simulink model "full_correlator"  (R2022a)
settings: Solver=VariableStepDiscrete  StartTime=0.0  StopTime=4000  RelTol=1e-3
libraries: hdlBasic x2638, hdlSSR x215, hdlDSPIP x4, xbsIndex_r4 x1, xps_library x1
(part 32 of 43)

== system full_correlator/Subsystem5/Vector Complex Mult2/Mult6 ==
  note: MULT2 and MULT3 settings
      | -------------------------------------
      | w mux = 0 op[8:7] = 00
      | z mux = C op[6:4] = 011
      | x mux = M op[3:2] = 01
      | y mux = M op[1:0] = 01
      | carryinsel = 000
      | inmode = bin2dec('00100') (D+B) vs bin2dec('01100') (D-B);
      | inmode[4]=0 for B2 selection; inmode[3]=0 preadd; inmode[0]=0 A2
      | alumode = bin2dec('0000') (Z+W+X+Y+CIN)
  note: latency = 6
  note: -(D-A)*B
  note: A*B
      | a = 30 bits
      | b = 18 bits,
      | d = 27 bits
  note: (A_re[25:0] + jA_im[25:0]) x (B_re[16:0] + jB_im[16:0])= Out_re[43:0] + jOut_im[43:0]
      | –Out_re[43:0]= ((A_re[25:0] x B_re[16:0]) - (A_im[25:0] x B_im[16:0]))
      | –Out_im[43:0]= ((A_re[25:0] x B_im[16:0]) + (A_im[25:0] x B_re[16:0]))
      |
      | Re-factored for three DSP slice version that uses PreAdders
      | –Out_re[43:0]= (CF) - ((B_re[16:0] – B_im[16:0]) x A_re[25:0])
      | –Out_im[43:0]= (CF) + ((B_re[16:0] + B_im[16:0]) x A_im[25:0])
      | Common factor that is shared
      | –CF=((A_re[25:0] – A_im[25:0]) x B_im[16:0])
  note: MULT1 settings
      | -------------------------------------
      | w mux = rnd op[8:7] = 00
      | z mux = C op[6:4] = 000
      | x mux = M op[3:2] = 01
      | y mux = M op[1:0] = 01
      | carryinsel = 000
      | inmode = bin2dec('01101') (D-A)
      | inmode[4]=0 for B2 selection; inmode[3]=0 preadd; inmode[0]=0 A2
      | alumode = bin2dec('0011') Z-(W+X+Y+CIN)
  note: (D-B)*A+C
  note: (D+B)*A+C
  A_re : Inport
  A_im : Inport  Port=2
  B_re : Inport  Port=3
  B_im : Inport  Port=4
  BitBasher : hdlBasic/BitBasher  bitexpr=out_44_40={in_48[43:0]}  display_expr=off  sr_1=out_44_40  arith_type1="Signed  (2's comp)"  bin_pt1=41  sr_2=2  arith_type2=Unsigned  bin_pt2=0  sr_3=3  arith_type3=Unsigned  bin_pt3=0  sr_4=4  arith_type4=Unsigned  bin_pt4=0  XmcBlockStatus=1  maskContainerNames=group1  block_type=bitbasher  block_config=sysgen:BitBasher_config
  BitBasher1 : hdlBasic/BitBasher  bitexpr=out_44_40={in_48[43:0]}  display_expr=off  sr_1=out_44_40  arith_type1="Signed  (2's comp)"  bin_pt1=41  sr_2=2  arith_type2=Unsigned  bin_pt2=0  sr_3=3  arith_type3=Unsigned  bin_pt3=0  sr_4=4  arith_type4=Unsigned  bin_pt4=0  XmcBlockStatus=1  maskContainerNames=group1  block_type=bitbasher  block_config=sysgen:BitBasher_config
  Constant10 : hdlBasic/Constant  const=bin2dec('000')  gui_display_data_type=Fixed-point  arith_type=Unsigned  n_bits=3  bin_pt=0  preci_type=Single  exp_width=8  frac_width=24  explicit_period=off  period=1  XmcBlockStatus=1  maskContainerNames=tabcontainer1  block_type=constant  block_config=sysgen:Constant_config
  Constant11 : hdlBasic/Constant  const=bin2dec('01101')  gui_display_data_type=Fixed-point  arith_type=Unsigned  n_bits=5  bin_pt=0  preci_type=Single  exp_width=8  frac_width=24  explicit_period=off  period=1  XmcBlockStatus=1  maskContainerNames=tabcontainer1  block_type=constant  block_config=sysgen:Constant_config
  Constant12 : hdlBasic/Constant  const=bin2dec('000000101')  gui_display_data_type=Fixed-point  arith_type=Unsigned  n_bits=9  bin_pt=0  preci_type=Single  exp_width=8  frac_width=24  explicit_period=off  period=1  XmcBlockStatus=1  maskContainerNames=tabcontainer1  block_type=constant  block_config=sysgen:Constant_config
  Constant13 : hdlBasic/Constant  const=0  gui_display_data_type=Fixed-point  arith_type=Unsigned  n_bits=1  bin_pt=0  preci_type=Single  exp_width=8  frac_width=24  explicit_period=off  period=1  XmcBlockStatus=1  maskContainerNames=tabcontainer1  block_type=constant  block_config=sysgen:Constant_config
  Constant14 : hdlBasic/Constant  const=0  gui_display_data_type=Fixed-point  arith_type=Unsigned  n_bits=1  bin_pt=0  preci_type=Single  exp_width=8  frac_width=24  explicit_period=off  period=1  XmcBlockStatus=1  maskContainerNames=tabcontainer1  block_type=constant  block_config=sysgen:Constant_config
  Constant15 : hdlBasic/Constant  const=bin2dec('000')  gui_display_data_type=Fixed-point  arith_type=Unsigned  n_bits=3  bin_pt=0  preci_type=Single  exp_width=8  frac_width=24  explicit_period=off  period=1  XmcBlockStatus=1  maskContainerNames=tabcontainer1  block_type=constant  block_config=sysgen:Constant_config
  Constant16 : hdlBasic/Constant  const=bin2dec('00100')  gui_display_data_type=Fixed-point  arith_type=Unsigned  n_bits=5  bin_pt=0  preci_type=Single  exp_width=8  frac_width=24  explicit_period=off  period=1  XmcBlockStatus=1  maskContainerNames=tabcontainer1  block_type=constant  block_config=sysgen:Constant_config
  Constant17 : hdlBasic/Constant  const=bin2dec('000110101')  gui_display_data_type=Fixed-point  arith_type=Unsigned  n_bits=9  bin_pt=0  preci_type=Single  exp_width=8  frac_width=24  explicit_period=off  period=1  XmcBlockStatus=1  maskContainerNames=tabcontainer1  block_type=constant  block_config=sysgen:Constant_config
  Constant18 : hdlBasic/Constant  const=bin2dec('0000')  gui_display_data_type=Fixed-point  arith_type=Unsigned  n_bits=4  bin_pt=0  preci_type=Single  exp_width=8  frac_width=24  explicit_period=off  period=1  XmcBlockStatus=1  maskContainerNames=tabcontainer1  block_type=constant  block_config=sysgen:Constant_config
  Constant4 : hdlBasic/Constant  const=bin2dec('000')  gui_display_data_type=Fixed-point  arith_type=Unsigned  n_bits=3  bin_pt=0  preci_type=Single  exp_width=8  frac_width=24  explicit_period=off  period=1  XmcBlockStatus=1  maskContainerNames=tabcontainer1  block_type=constant  block_config=sysgen:Constant_config
  Constant5 : hdlBasic/Constant  const=bin2dec('01100')  gui_display_data_type=Fixed-point  arith_type=Unsigned  n_bits=5  bin_pt=0  preci_type=Single  exp_width=8  frac_width=24  explicit_period=off  period=1  XmcBlockStatus=1  maskContainerNames=tabcontainer1  block_type=constant  block_config=sysgen:Constant_config
  Constant6 : hdlBasic/Constant  const=bin2dec('000110101')  gui_display_data_type=Fixed-point  arith_type=Unsigned  n_bits=9  bin_pt=0  preci_type=Single  exp_width=8  frac_width=24  explicit_period=off  period=1  XmcBlockStatus=1  maskContainerNames=tabcontainer1  block_type=constant  block_config=sysgen:Constant_config
  Constant7 : hdlBasic/Constant  const=bin2dec('0000')  gui_display_data_type=Fixed-point  arith_type=Unsigned  n_bits=4  bin_pt=0  preci_type=Single  exp_width=8  frac_width=24  explicit_period=off  period=1  XmcBlockStatus=1  maskContainerNames=tabcontainer1  block_type=constant  block_config=sysgen:Constant_config
  Constant8 : hdlBasic/Constant  const=bin2dec('0011')  gui_display_data_type=Fixed-point  arith_type=Unsigned  n_bits=4  bin_pt=0  preci_type=Single  exp_width=8  frac_width=24  explicit_period=off  period=1  XmcBlockStatus=1  maskContainerNames=tabcontainer1  block_type=constant  block_config=sysgen:Constant_config
  Constant9 : hdlBasic/Constant  const=0  gui_display_data_type=Fixed-point  arith_type=Unsigned  n_bits=1  bin_pt=0  preci_type=Single  exp_width=8  frac_width=24  explicit_period=off  period=1  XmcBlockStatus=1  maskContainerNames=tabcontainer1  block_type=constant  block_config=sysgen:Constant_config
  Delay : hdlBasic/Delay  rst=off  en=off  latency=2  reg_retiming=off  XmcBlockStatus=1  maskContainerNames=group1  block_type=delay  block_config=sysgen:Delay_config
  Delay1 : hdlBasic/Delay  rst=off  en=off  latency=2  reg_retiming=off  XmcBlockStatus=1  maskContainerNames=group1  block_type=delay  block_config=sysgen:Delay_config
  MULT1 : hdlBasic/DSP48E2   use_a=Direct from a port  use_b=Direct from b port  addsub_mode=One 48-bit Unit  xl_useadderonly=off  xl_dynamicmult=off  preaddinsel=A  amultsel=AD  bmultsel=B  enable_d=on  reset_preg=off  auto_reset_pr=RESET  pattern_from_creg=Pattern Input from c port  pattern='000000000000'  mask_from_creg=Mask Input from c port  pattern_mask='000000000000'  rnd='000000000000'  widexor=off  xormode=XOR12  use_op=off  use_creg=off  rst_all=off  en_all=off  use_pcin=off  use_carrycascin=off  use_multsignin=off  use_carryout=off  use_patterndetect=off  use_patternbdetect=off  use_overflow=off  use_underflow=off  use_acout=on  use_bcout=on  use_pcout=off  use_multsignout=off  use_carrycascout=off  pipeline_a=2  pipeline_b=2  pipeline_acout=2  pipeline_bcout=1  pipeline_c=on  pipeline_p=on  pipeline_mult=on  pipeline_opmode=off  pipeline_alumode=off  pipeline_carryin=off  pipeline_carryinsel=off  dreg=on  adreg=on  register_inmode=off  rst_a=off  rst_b=off  rst_c=off  rst_mult=off  rst_p=off  rst_carry_in=off  rst_alumode=off  rst_ctrl=off  reset_port_d=off  reset_port_inmode=off  en_a1=off  en_a2=off  en_b1=off  en_b2=off  en_c=off  en_mult=off  en_p=off  en_carry_in=off  en_alumode=off  en_multcarryin=off  en_ctrl=off  enable_port_regd=off  enable_port_regad=off  enable_port_reginmode=off  alumode_inverted=off  alumode_inverted_value='0000'  is_carryin_inverted=off  inmode_inverted=off  inmode_inverted_value='00000'  opmode_inverted=off  opmode_inverted_value='000000000'  is_rstallcarryin_inverted=off  is_rstalumode_inverted=off  is_rsta_inverted=off  is_rstb_inverted=off  is_rstc_inverted=off  is_rstd_inverted=off  is_rstctrl_inverted=off  is_rstinmode_inverted=off  is_rstm_inverted=off  is_rstp_inverted=off  use_synth_model=off  simulation_type=fast_sim  is_clk_inverted=false  XmcBlockStatus=1  maskContainerNames=tabcontainer1  block_type=dsp48e2  block_config=sysgen:DSP48E2_config  block_height=1080  block_width=800
  MULT2 : hdlBasic/DSP48E2   use_a=Cascaded from acin port  use_b=Cascaded from bcin port  addsub_mode=One 48-bit Unit  xl_useadderonly=off  xl_dynamicmult=off  preaddinsel=B  amultsel=A  bmultsel=AD  enable_d=on  reset_preg=off  auto_reset_pr=RESET  pattern_from_creg=Pattern Input from c port  pattern='000000000000'  mask_from_creg=Mask Input from c port  pattern_mask='000000000000'  rnd='000000000000'  widexor=off  xormode=XOR12  use_op=off  use_creg=on  rst_all=off  en_all=off  use_pcin=off  use_carrycascin=off  use_multsignin=off  use_carryout=off  use_patterndetect=off  use_patternbdetect=off  use_overflow=off  use_underflow=off  use_acout=off  use_bcout=on  use_pcout=off  use_multsignout=off  use_carrycascout=off  pipeline_a=2  pipeline_b=2  pipeline_acout=1  pipeline_bcout=1  pipeline_c=on  pipeline_p=on  pipeline_mult=on  pipeline_opmode=off  pipeline_alumode=off  pipeline_carryin=off  pipeline_carryinsel=off  dreg=on  adreg=on  register_inmode=off  rst_a=off  rst_b=off  rst_c=off  rst_mult=off  rst_p=off  rst_carry_in=off  rst_alumode=off  rst_ctrl=off  reset_port_d=off  reset_port_inmode=off  en_a1=off  en_a2=off  en_b1=off  en_b2=off  en_c=off  en_mult=off  en_p=off  en_carry_in=off  en_alumode=off  en_multcarryin=off  en_ctrl=off  enable_port_regd=off  enable_port_regad=off  enable_port_reginmode=off  alumode_inverted=off  alumode_inverted_value='0000'  is_carryin_inverted=off  inmode_inverted=off  inmode_inverted_value='00000'  opmode_inverted=off  opmode_inverted_value='000000000'  is_rstallcarryin_inverted=off  is_rstalumode_inverted=off  is_rsta_inverted=off  is_rstb_inverted=off  is_rstc_inverted=off  is_rstd_inverted=off  is_rstctrl_inverted=off  is_rstinmode_inverted=off  is_rstm_inverted=off  is_rstp_inverted=off  use_synth_model=off  simulation_type=fast_sim  is_clk_inverted=false  XmcBlockStatus=1  maskContainerNames=tabcontainer1  block_type=dsp48e2  block_config=sysgen:DSP48E2_config  block_height=1080  block_width=800
  MULT3 : hdlBasic/DSP48E2   use_a=Direct from a port  use_b=Cascaded from bcin port  addsub_mode=One 48-bit Unit  xl_useadderonly=off  xl_dynamicmult=off  preaddinsel=B  amultsel=A  bmultsel=AD  enable_d=on  reset_preg=off  auto_reset_pr=RESET  pattern_from_creg=Pattern Input from c port  pattern='000000000000'  mask_from_creg=Mask Input from c port  pattern_mask='000000000000'  rnd='000000000000'  widexor=off  xormode=XOR12  use_op=off  use_creg=on  rst_all=off  en_all=off  use_pcin=off  use_carrycascin=off  use_multsignin=off  use_carryout=off  use_patterndetect=off  use_patternbdetect=off  use_overflow=off  use_underflow=off  use_acout=off  use_bcout=off  use_pcout=off  use_multsignout=off  use_carrycascout=off  pipeline_a=2  pipeline_b=1  pipeline_acout=1  pipeline_bcout=1  pipeline_c=on  pipeline_p=on  pipeline_mult=on  pipeline_opmode=off  pipeline_alumode=off  pipeline_carryin=off  pipeline_carryinsel=off  dreg=on  adreg=on  register_inmode=off  rst_a=off  rst_b=off  rst_c=off  rst_mult=off  rst_p=off  rst_carry_in=off  rst_alumode=off  rst_ctrl=off  reset_port_d=off  reset_port_inmode=off  en_a1=off  en_a2=off  en_b1=off  en_b2=off  en_c=off  en_mult=off  en_p=off  en_carry_in=off  en_alumode=off  en_multcarryin=off  en_ctrl=off  enable_port_regd=off  enable_port_regad=off  enable_port_reginmode=off  alumode_inverted=off  alumode_inverted_value='0000'  is_carryin_inverted=off  inmode_inverted=off  inmode_inverted_value='00000'  opmode_inverted=off  opmode_inverted_value='000000000'  is_rstallcarryin_inverted=off  is_rstalumode_inverted=off  is_rsta_inverted=off  is_rstb_inverted=off  is_rstc_inverted=off  is_rstd_inverted=off  is_rstctrl_inverted=off  is_rstinmode_inverted=off  is_rstm_inverted=off  is_rstp_inverted=off  use_synth_model=off  simulation_type=fast_sim  is_clk_inverted=false  XmcBlockStatus=1  maskContainerNames=tabcontainer1  block_type=dsp48e2  block_config=sysgen:DSP48E2_config  block_height=1080  block_width=800
  bit_bash1 : hdlBasic/BitBasher  bitexpr=ao={ain[25],ain[25:0]} % sign extend to 27 bits  display_expr=off  sr_1=ao  arith_type1="Signed  (2's comp)"  bin_pt1=0  sr_2=a_dsp48  arith_type2="Signed  (2's comp)"  bin_pt2=0  sr_3=p2  arith_type3=Unsigned  bin_pt3=0  sr_4=4  arith_type4=Unsigned  bin_pt4=0  XmcBlockStatus=1  maskContainerNames=group1  block_type=bitbasher  block_config=sysgen:BitBasher_config
  bit_bash2 : hdlBasic/BitBasher  bitexpr=ao={4{ain[25]},ain[25:0]} % sign extend to 30 bits  display_expr=off  sr_1=ao  arith_type1="Signed  (2's comp)"  bin_pt1=0  sr_2=a_dsp48  arith_type2="Signed  (2's comp)"  bin_pt2=0  sr_3=p2  arith_type3=Unsigned  bin_pt3=0  sr_4=4  arith_type4=Unsigned  bin_pt4=0  XmcBlockStatus=1  maskContainerNames=group1  block_type=bitbasher  block_config=sysgen:BitBasher_config
  bit_bash3 : hdlBasic/BitBasher  bitexpr=bo={ bin[16] , bin[16:0] }; % sign extend to 18 bit data  display_expr=off  sr_1=bo  arith_type1="Signed  (2's comp)"  bin_pt1=0  sr_2=b_dsp48  arith_type2="Signed  (2's comp)"  bin_pt2=0  sr_3=p2  arith_type3=Unsigned  bin_pt3=0  sr_4=4  arith_type4=Unsigned  bin_pt4=0  XmcBlockStatus=1  maskContainerNames=group1  block_type=bitbasher  block_config=sysgen:BitBasher_config
  bit_bash4 : hdlBasic/BitBasher  bitexpr=bo={ 10{bin[16]} , bin[16:0] }; % sign extend to 27 bit data  display_expr=off  sr_1=bo  arith_type1="Signed  (2's comp)"  bin_pt1=0  sr_2=b_dsp48  arith_type2="Signed  (2's comp)"  bin_pt2=0  sr_3=p2  arith_type3=Unsigned  bin_pt3=0  sr_4=4  arith_type4=Unsigned  bin_pt4=0  XmcBlockStatus=1  maskContainerNames=group1  block_type=bitbasher  block_config=sysgen:BitBasher_config
  bit_bash8 : hdlBasic/BitBasher  bitexpr=ao={3{ain[26]},ain[26:0]} % sign extend to 30 bits  display_expr=off  sr_1=ao  arith_type1="Signed  (2's comp)"  bin_pt1=0  sr_2=a_dsp48  arith_type2="Signed  (2's comp)"  bin_pt2=0  sr_3=p2  arith_type3=Unsigned  bin_pt3=0  sr_4=4  arith_type4=Unsigned  bin_pt4=0  XmcBlockStatus=1  maskContainerNames=group1  block_type=bitbasher  block_config=sysgen:BitBasher_config
  C_re : Outport  VectorParamsAs1DForOutWhenUnconnected=off
  C_im : Outport  Port=2  VectorParamsAs1DForOutWhenUnconnected=off
  wires:
  BitBasher1/1 -> C_re/1  "C_re"
  MULT3/1 -> BitBasher/1
  Delay/1 -> MULT3/4, MULT2/4  "B_re_int_dly2"
  Constant15/1 -> MULT3/8
  MULT1/3 -> MULT2/2  "bcout_MULT1"
  Constant7/1 -> MULT2/6
  Constant13/1 -> MULT2/7
  Constant4/1 -> MULT2/8
  Constant5/1 -> MULT2/9
  Constant8/1 -> MULT1/5
  Constant9/1 -> MULT1/6
  Delay1/1 -> MULT3/1  "A_im_int_dly2"
  bit_bash4/1 -> Delay/1  "B_re_int"
  bit_bash8/1 -> Delay1/1
  Constant6/1 -> MULT2/5
  MULT2/2 -> MULT3/2  "bcout_MULT2"
  Constant18/1 -> MULT3/6
  Constant11/1 -> MULT1/8
  Constant12/1 -> MULT1/4
  Constant10/1 -> MULT1/7
  MULT1/2 -> MULT2/1  "acout_MULT1"
  MULT2/1 -> BitBasher1/1  "out_re"
  Constant16/1 -> MULT3/9
  Constant14/1 -> MULT3/7
  Constant17/1 -> MULT3/5
  A_im/1 -> bit_bash1/1
  B_im/1 -> bit_bash3/1
  A_re/1 -> bit_bash2/1
  MULT1/1 -> MULT3/3, MULT2/3  "common"
  bit_bash1/1 -> bit_bash8/1, MULT1/3  "A_im_int"
  bit_bash2/1 -> MULT1/1  "A_re_int"
  bit_bash3/1 -> MULT1/2  "B_im_int"
  B_re/1 -> bit_bash4/1
  BitBasher/1 -> C_im/1  "C_im"

== system full_correlator/Subsystem5/Vector Complex Mult2/Mult7 ==
  note: MULT2 and MULT3 settings
      | -------------------------------------
      | w mux = 0 op[8:7] = 00
      | z mux = C op[6:4] = 011
      | x mux = M op[3:2] = 01
      | y mux = M op[1:0] = 01
      | carryinsel = 000
      | inmode = bin2dec('00100') (D+B) vs bin2dec('01100') (D-B);
      | inmode[4]=0 for B2 selection; inmode[3]=0 preadd; inmode[0]=0 A2
      | alumode = bin2dec('0000') (Z+W+X+Y+CIN)
  note: latency = 6
  note: -(D-A)*B
  note: A*B
      | a = 30 bits
      | b = 18 bits,
      | d = 27 bits
  note: (A_re[25:0] + jA_im[25:0]) x (B_re[16:0] + jB_im[16:0])= Out_re[43:0] + jOut_im[43:0]
      | –Out_re[43:0]= ((A_re[25:0] x B_re[16:0]) - (A_im[25:0] x B_im[16:0]))
      | –Out_im[43:0]= ((A_re[25:0] x B_im[16:0]) + (A_im[25:0] x B_re[16:0]))
      |
      | Re-factored for three DSP slice version that uses PreAdders
      | –Out_re[43:0]= (CF) - ((B_re[16:0] – B_im[16:0]) x A_re[25:0])
      | –Out_im[43:0]= (CF) + ((B_re[16:0] + B_im[16:0]) x A_im[25:0])
      | Common factor that is shared
      | –CF=((A_re[25:0] – A_im[25:0]) x B_im[16:0])
  note: MULT1 settings
      | -------------------------------------
      | w mux = rnd op[8:7] = 00
      | z mux = C op[6:4] = 000
      | x mux = M op[3:2] = 01
      | y mux = M op[1:0] = 01
      | carryinsel = 000
      | inmode = bin2dec('01101') (D-A)
      | inmode[4]=0 for B2 selection; inmode[3]=0 preadd; inmode[0]=0 A2
      | alumode = bin2dec('0011') Z-(W+X+Y+CIN)
  note: (D-B)*A+C
  note: (D+B)*A+C
  A_re : Inport
  A_im : Inport  Port=2
  B_re : Inport  Port=3
  B_im : Inport  Port=4
  BitBasher : hdlBasic/BitBasher  bitexpr=out_44_40={in_48[43:0]}  display_expr=off  sr_1=out_44_40  arith_type1="Signed  (2's comp)"  bin_pt1=41  sr_2=2  arith_type2=Unsigned  bin_pt2=0  sr_3=3  arith_type3=Unsigned  bin_pt3=0  sr_4=4  arith_type4=Unsigned  bin_pt4=0  XmcBlockStatus=1  maskContainerNames=group1  block_type=bitbasher  block_config=sysgen:BitBasher_config
  BitBasher1 : hdlBasic/BitBasher  bitexpr=out_44_40={in_48[43:0]}  display_expr=off  sr_1=out_44_40  arith_type1="Signed  (2's comp)"  bin_pt1=41  sr_2=2  arith_type2=Unsigned  bin_pt2=0  sr_3=3  arith_type3=Unsigned  bin_pt3=0  sr_4=4  arith_type4=Unsigned  bin_pt4=0  XmcBlockStatus=1  maskContainerNames=group1  block_type=bitbasher  block_config=sysgen:BitBasher_config
  Constant10 : hdlBasic/Constant  const=bin2dec('000')  gui_display_data_type=Fixed-point  arith_type=Unsigned  n_bits=3  bin_pt=0  preci_type=Single  exp_width=8  frac_width=24  explicit_period=off  period=1  XmcBlockStatus=1  maskContainerNames=tabcontainer1  block_type=constant  block_config=sysgen:Constant_config
  Constant11 : hdlBasic/Constant  const=bin2dec('01101')  gui_display_data_type=Fixed-point  arith_type=Unsigned  n_bits=5  bin_pt=0  preci_type=Single  exp_width=8  frac_width=24  explicit_period=off  period=1  XmcBlockStatus=1  maskContainerNames=tabcontainer1  block_type=constant  block_config=sysgen:Constant_config
  Constant12 : hdlBasic/Constant  const=bin2dec('000000101')  gui_display_data_type=Fixed-point  arith_type=Unsigned  n_bits=9  bin_pt=0  preci_type=Single  exp_width=8  frac_width=24  explicit_period=off  period=1  XmcBlockStatus=1  maskContainerNames=tabcontainer1  block_type=constant  block_config=sysgen:Constant_config
  Constant13 : hdlBasic/Constant  const=0  gui_display_data_type=Fixed-point  arith_type=Unsigned  n_bits=1  bin_pt=0  preci_type=Single  exp_width=8  frac_width=24  explicit_period=off  period=1  XmcBlockStatus=1  maskContainerNames=tabcontainer1  block_type=constant  block_config=sysgen:Constant_config
  Constant14 : hdlBasic/Constant  const=0  gui_display_data_type=Fixed-point  arith_type=Unsigned  n_bits=1  bin_pt=0  preci_type=Single  exp_width=8  frac_width=24  explicit_period=off  period=1  XmcBlockStatus=1  maskContainerNames=tabcontainer1  block_type=constant  block_config=sysgen:Constant_config
  Constant15 : hdlBasic/Constant  const=bin2dec('000')  gui_display_data_type=Fixed-point  arith_type=Unsigned  n_bits=3  bin_pt=0  preci_type=Single  exp_width=8  frac_width=24  explicit_period=off  period=1  XmcBlockStatus=1  maskContainerNames=tabcontainer1  block_type=constant  block_config=sysgen:Constant_config
  Constant16 : hdlBasic/Constant  const=bin2dec('00100')  gui_display_data_type=Fixed-point  arith_type=Unsigned  n_bits=5  bin_pt=0  preci_type=Single  exp_width=8  frac_width=24  explicit_period=off  period=1  XmcBlockStatus=1  maskContainerNames=tabcontainer1  block_type=constant  block_config=sysgen:Constant_config
  Constant17 : hdlBasic/Constant  const=bin2dec('000110101')  gui_display_data_type=Fixed-point  arith_type=Unsigned  n_bits=9  bin_pt=0  preci_type=Single  exp_width=8  frac_width=24  explicit_period=off  period=1  XmcBlockStatus=1  maskContainerNames=tabcontainer1  block_type=constant  block_config=sysgen:Constant_config
  Constant18 : hdlBasic/Constant  const=bin2dec('0000')  gui_display_data_type=Fixed-point  arith_type=Unsigned  n_bits=4  bin_pt=0  preci_type=Single  exp_width=8  frac_width=24  explicit_period=off  period=1  XmcBlockStatus=1  maskContainerNames=tabcontainer1  block_type=constant  block_config=sysgen:Constant_config
  Constant4 : hdlBasic/Constant  const=bin2dec('000')  gui_display_data_type=Fixed-point  arith_type=Unsigned  n_bits=3  bin_pt=0  preci_type=Single  exp_width=8  frac_width=24  explicit_period=off  period=1  XmcBlockStatus=1  maskContainerNames=tabcontainer1  block_type=constant  block_config=sysgen:Constant_config
  Constant5 : hdlBasic/Constant  const=bin2dec('01100')  gui_display_data_type=Fixed-point  arith_type=Unsigned  n_bits=5  bin_pt=0  preci_type=Single  exp_width=8  frac_width=24  explicit_period=off  period=1  XmcBlockStatus=1  maskContainerNames=tabcontainer1  block_type=constant  block_config=sysgen:Constant_config
  Constant6 : hdlBasic/Constant  const=bin2dec('000110101')  gui_display_data_type=Fixed-point  arith_type=Unsigned  n_bits=9  bin_pt=0  preci_type=Single  exp_width=8  frac_width=24  explicit_period=off  period=1  XmcBlockStatus=1  maskContainerNames=tabcontainer1  block_type=constant  block_config=sysgen:Constant_config
  Constant7 : hdlBasic/Constant  const=bin2dec('0000')  gui_display_data_type=Fixed-point  arith_type=Unsigned  n_bits=4  bin_pt=0  preci_type=Single  exp_width=8  frac_width=24  explicit_period=off  period=1  XmcBlockStatus=1  maskContainerNames=tabcontainer1  block_type=constant  block_config=sysgen:Constant_config
  Constant8 : hdlBasic/Constant  const=bin2dec('0011')  gui_display_data_type=Fixed-point  arith_type=Unsigned  n_bits=4  bin_pt=0  preci_type=Single  exp_width=8  frac_width=24  explicit_period=off  period=1  XmcBlockStatus=1  maskContainerNames=tabcontainer1  block_type=constant  block_config=sysgen:Constant_config
  Constant9 : hdlBasic/Constant  const=0  gui_display_data_type=Fixed-point  arith_type=Unsigned  n_bits=1  bin_pt=0  preci_type=Single  exp_width=8  frac_width=24  explicit_period=off  period=1  XmcBlockStatus=1  maskContainerNames=tabcontainer1  block_type=constant  block_config=sysgen:Constant_config
  Delay : hdlBasic/Delay  rst=off  en=off  latency=2  reg_retiming=off  XmcBlockStatus=1  maskContainerNames=group1  block_type=delay  block_config=sysgen:Delay_config
  Delay1 : hdlBasic/Delay  rst=off  en=off  latency=2  reg_retiming=off  XmcBlockStatus=1  maskContainerNames=group1  block_type=delay  block_config=sysgen:Delay_config
  MULT1 : hdlBasic/DSP48E2   use_a=Direct from a port  use_b=Direct from b port  addsub_mode=One 48-bit Unit  xl_useadderonly=off  xl_dynamicmult=off  preaddinsel=A  amultsel=AD  bmultsel=B  enable_d=on  reset_preg=off  auto_reset_pr=RESET  pattern_from_creg=Pattern Input from c port  pattern='000000000000'  mask_from_creg=Mask Input from c port  pattern_mask='000000000000'  rnd='000000000000'  widexor=off  xormode=XOR12  use_op=off  use_creg=off  rst_all=off  en_all=off  use_pcin=off  use_carrycascin=off  use_multsignin=off  use_carryout=off  use_patterndetect=off  use_patternbdetect=off  use_overflow=off  use_underflow=off  use_acout=on  use_bcout=on  use_pcout=off  use_multsignout=off  use_carrycascout=off  pipeline_a=2  pipeline_b=2  pipeline_acout=2  pipeline_bcout=1  pipeline_c=on  pipeline_p=on  pipeline_mult=on  pipeline_opmode=off  pipeline_alumode=off  pipeline_carryin=off  pipeline_carryinsel=off  dreg=on  adreg=on  register_inmode=off  rst_a=off  rst_b=off  rst_c=off  rst_mult=off  rst_p=off  rst_carry_in=off  rst_alumode=off  rst_ctrl=off  reset_port_d=off  reset_port_inmode=off  en_a1=off  en_a2=off  en_b1=off  en_b2=off  en_c=off  en_mult=off  en_p=off  en_carry_in=off  en_alumode=off  en_multcarryin=off  en_ctrl=off  enable_port_regd=off  enable_port_regad=off  enable_port_reginmode=off  alumode_inverted=off  alumode_inverted_value='0000'  is_carryin_inverted=off  inmode_inverted=off  inmode_inverted_value='00000'  opmode_inverted=off  opmode_inverted_value='000000000'  is_rstallcarryin_inverted=off  is_rstalumode_inverted=off  is_rsta_inverted=off  is_rstb_inverted=off  is_rstc_inverted=off  is_rstd_inverted=off  is_rstctrl_inverted=off  is_rstinmode_inverted=off  is_rstm_inverted=off  is_rstp_inverted=off  use_synth_model=off  simulation_type=fast_sim  is_clk_inverted=false  XmcBlockStatus=1  maskContainerNames=tabcontainer1  block_type=dsp48e2  block_config=sysgen:DSP48E2_config  block_height=1080  block_width=800
  MULT2 : hdlBasic/DSP48E2   use_a=Cascaded from acin port  use_b=Cascaded from bcin port  addsub_mode=One 48-bit Unit  xl_useadderonly=off  xl_dynamicmult=off  preaddinsel=B  amultsel=A  bmultsel=AD  enable_d=on  reset_preg=off  auto_reset_pr=RESET  pattern_from_creg=Pattern Input from c port  pattern='000000000000'  mask_from_creg=Mask Input from c port  pattern_mask='000000000000'  rnd='000000000000'  widexor=off  xormode=XOR12  use_op=off  use_creg=on  rst_all=off  en_all=off  use_pcin=off  use_carrycascin=off  use_multsignin=off  use_carryout=off  use_patterndetect=off  use_patternbdetect=off  use_overflow=off  use_underflow=off  use_acout=off  use_bcout=on  use_pcout=off  use_multsignout=off  use_carrycascout=off  pipeline_a=2  pipeline_b=2  pipeline_acout=1  pipeline_bcout=1  pipeline_c=on  pipeline_p=on  pipeline_mult=on  pipeline_opmode=off  pipeline_alumode=off  pipeline_carryin=off  pipeline_carryinsel=off  dreg=on  adreg=on  register_inmode=off  rst_a=off  rst_b=off  rst_c=off  rst_mult=off  rst_p=off  rst_carry_in=off  rst_alumode=off  rst_ctrl=off  reset_port_d=off  reset_port_inmode=off  en_a1=off  en_a2=off  en_b1=off  en_b2=off  en_c=off  en_mult=off  en_p=off  en_carry_in=off  en_alumode=off  en_multcarryin=off  en_ctrl=off  enable_port_regd=off  enable_port_regad=off  enable_port_reginmode=off  alumode_inverted=off  alumode_inverted_value='0000'  is_carryin_inverted=off  inmode_inverted=off  inmode_inverted_value='00000'  opmode_inverted=off  opmode_inverted_value='000000000'  is_rstallcarryin_inverted=off  is_rstalumode_inverted=off  is_rsta_inverted=off  is_rstb_inverted=off  is_rstc_inverted=off  is_rstd_inverted=off  is_rstctrl_inverted=off  is_rstinmode_inverted=off  is_rstm_inverted=off  is_rstp_inverted=off  use_synth_model=off  simulation_type=fast_sim  is_clk_inverted=false  XmcBlockStatus=1  maskContainerNames=tabcontainer1  block_type=dsp48e2  block_config=sysgen:DSP48E2_config  block_height=1080  block_width=800
  MULT3 : hdlBasic/DSP48E2   use_a=Direct from a port  use_b=Cascaded from bcin port  addsub_mode=One 48-bit Unit  xl_useadderonly=off  xl_dynamicmult=off  preaddinsel=B  amultsel=A  bmultsel=AD  enable_d=on  reset_preg=off  auto_reset_pr=RESET  pattern_from_creg=Pattern Input from c port  pattern='000000000000'  mask_from_creg=Mask Input from c port  pattern_mask='000000000000'  rnd='000000000000'  widexor=off  xormode=XOR12  use_op=off  use_creg=on  rst_all=off  en_all=off  use_pcin=off  use_carrycascin=off  use_multsignin=off  use_carryout=off  use_patterndetect=off  use_patternbdetect=off  use_overflow=off  use_underflow=off  use_acout=off  use_bcout=off  use_pcout=off  use_multsignout=off  use_carrycascout=off  pipeline_a=2  pipeline_b=1  pipeline_acout=1  pipeline_bcout=1  pipeline_c=on  pipeline_p=on  pipeline_mult=on  pipeline_opmode=off  pipeline_alumode=off  pipeline_carryin=off  pipeline_carryinsel=off  dreg=on  adreg=on  register_inmode=off  rst_a=off  rst_b=off  rst_c=off  rst_mult=off  rst_p=off  rst_carry_in=off  rst_alumode=off  rst_ctrl=off  reset_port_d=off  reset_port_inmode=off  en_a1=off  en_a2=off  en_b1=off  en_b2=off  en_c=off  en_mult=off  en_p=off  en_carry_in=off  en_alumode=off  en_multcarryin=off  en_ctrl=off  enable_port_regd=off  enable_port_regad=off  enable_port_reginmode=off  alumode_inverted=off  alumode_inverted_value='0000'  is_carryin_inverted=off  inmode_inverted=off  inmode_inverted_value='00000'  opmode_inverted=off  opmode_inverted_value='000000000'  is_rstallcarryin_inverted=off  is_rstalumode_inverted=off  is_rsta_inverted=off  is_rstb_inverted=off  is_rstc_inverted=off  is_rstd_inverted=off  is_rstctrl_inverted=off  is_rstinmode_inverted=off  is_rstm_inverted=off  is_rstp_inverted=off  use_synth_model=off  simulation_type=fast_sim  is_clk_inverted=false  XmcBlockStatus=1  maskContainerNames=tabcontainer1  block_type=dsp48e2  block_config=sysgen:DSP48E2_config  block_height=1080  block_width=800
  bit_bash1 : hdlBasic/BitBasher  bitexpr=ao={ain[25],ain[25:0]} % sign extend to 27 bits  display_expr=off  sr_1=ao  arith_type1="Signed  (2's comp)"  bin_pt1=0  sr_2=a_dsp48  arith_type2="Signed  (2's comp)"  bin_pt2=0  sr_3=p2  arith_type3=Unsigned  bin_pt3=0  sr_4=4  arith_type4=Unsigned  bin_pt4=0  XmcBlockStatus=1  maskContainerNames=group1  block_type=bitbasher  block_config=sysgen:BitBasher_config
  bit_bash2 : hdlBasic/BitBasher  bitexpr=ao={4{ain[25]},ain[25:0]} % sign extend to 30 bits  display_expr=off  sr_1=ao  arith_type1="Signed  (2's comp)"  bin_pt1=0  sr_2=a_dsp48  arith_type2="Signed  (2's comp)"  bin_pt2=0  sr_3=p2  arith_type3=Unsigned  bin_pt3=0  sr_4=4  arith_type4=Unsigned  bin_pt4=0  XmcBlockStatus=1  maskContainerNames=group1  block_type=bitbasher  block_config=sysgen:BitBasher_config
  bit_bash3 : hdlBasic/BitBasher  bitexpr=bo={ bin[16] , bin[16:0] }; % sign extend to 18 bit data  display_expr=off  sr_1=bo  arith_type1="Signed  (2's comp)"  bin_pt1=0  sr_2=b_dsp48  arith_type2="Signed  (2's comp)"  bin_pt2=0  sr_3=p2  arith_type3=Unsigned  bin_pt3=0  sr_4=4  arith_type4=Unsigned  bin_pt4=0  XmcBlockStatus=1  maskContainerNames=group1  block_type=bitbasher  block_config=sysgen:BitBasher_config
  bit_bash4 : hdlBasic/BitBasher  bitexpr=bo={ 10{bin[16]} , bin[16:0] }; % sign extend to 27 bit data  display_expr=off  sr_1=bo  arith_type1="Signed  (2's comp)"  bin_pt1=0  sr_2=b_dsp48  arith_type2="Signed  (2's comp)"  bin_pt2=0  sr_3=p2  arith_type3=Unsigned  bin_pt3=0  sr_4=4  arith_type4=Unsigned  bin_pt4=0  XmcBlockStatus=1  maskContainerNames=group1  block_type=bitbasher  block_config=sysgen:BitBasher_config
  bit_bash8 : hdlBasic/BitBasher  bitexpr=ao={3{ain[26]},ain[26:0]} % sign extend to 30 bits  display_expr=off  sr_1=ao  arith_type1="Signed  (2's comp)"  bin_pt1=0  sr_2=a_dsp48  arith_type2="Signed  (2's comp)"  bin_pt2=0  sr_3=p2  arith_type3=Unsigned  bin_pt3=0  sr_4=4  arith_type4=Unsigned  bin_pt4=0  XmcBlockStatus=1  maskContainerNames=group1  block_type=bitbasher  block_config=sysgen:BitBasher_config
  C_re : Outport  VectorParamsAs1DForOutWhenUnconnected=off
  C_im : Outport  Port=2  VectorParamsAs1DForOutWhenUnconnected=off
  wires:
  BitBasher1/1 -> C_re/1  "C_re"
  MULT3/1 -> BitBasher/1
  Delay/1 -> MULT3/4, MULT2/4  "B_re_int_dly2"
  Constant15/1 -> MULT3/8
  MULT1/3 -> MULT2/2  "bcout_MULT1"
  Constant7/1 -> MULT2/6
  Constant13/1 -> MULT2/7
  Constant4/1 -> MULT2/8
  Constant5/1 -> MULT2/9
  Constant8/1 -> MULT1/5
  Constant9/1 -> MULT1/6
  Delay1/1 -> MULT3/1  "A_im_int_dly2"
  bit_bash4/1 -> Delay/1  "B_re_int"
  bit_bash8/1 -> Delay1/1
  Constant6/1 -> MULT2/5
  MULT2/2 -> MULT3/2  "bcout_MULT2"
  Constant18/1 -> MULT3/6
  Constant11/1 -> MULT1/8
  Constant12/1 -> MULT1/4
  Constant10/1 -> MULT1/7
  MULT1/2 -> MULT2/1  "acout_MULT1"
  MULT2/1 -> BitBasher1/1  "out_re"
  Constant16/1 -> MULT3/9
  Constant14/1 -> MULT3/7
  Constant17/1 -> MULT3/5
  A_im/1 -> bit_bash1/1
  B_im/1 -> bit_bash3/1
  A_re/1 -> bit_bash2/1
  MULT1/1 -> MULT3/3, MULT2/3  "common"
  bit_bash1/1 -> bit_bash8/1, MULT1/3  "A_im_int"
  bit_bash2/1 -> MULT1/1  "A_re_int"
  bit_bash3/1 -> MULT1/2  "B_im_int"
  B_re/1 -> bit_bash4/1
  BitBasher/1 -> C_im/1  "C_im"
